simulink model "LQI_example"  (R2023b)
settings: Solver=ode8  StartTime=0.0  StopTime=5  FixedStep=0.04  RelTol=1e-3
values from neighbouring files (symbols this model uses):
  A = [0 1; -2 -3]    [LQI_servo_Example.m]
  B = [0; 1]    [LQI_servo_Example.m]
  K_lqi = lqi( plant, Q, R)    [LQI_servo_Example.m]
settings Model: Creator=afons  LastModifiedBy=afons

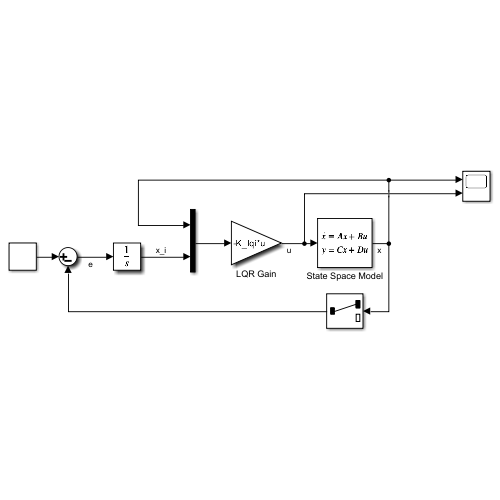
[thumbnail: Simulink's stored preview of the top-level diagram]
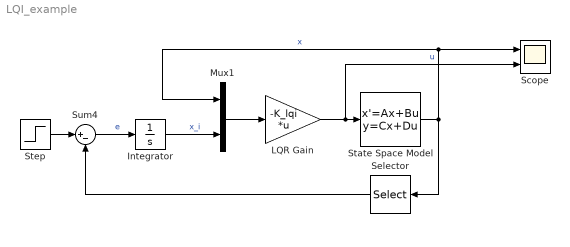
== system LQI_example ==
  Integrator : Integrator
  LQR Gain : Gain  Gain=-K_lqi  Multiplication=Matrix(K*u)  SaturateOnIntegerOverflow=on  OutDataTypeStr=Inherit: Same as input  ParamDataTypeStr=Inherit: Same as input
  Mux1 : Mux  Inputs=2
  Scope : Scope  NumInputPorts=2
  Selector : Selector  InputPortWidth=2  IndexOptions=Index vector (dialog)  Indices=1  OutputSizes=1
  State Space Model : StateSpace  A=A  B=B  C=eye(2)  D=zeros(2,1)  InitialCondition=0
  Step : Step  Time=0  SampleTime=0
  Sum4 : Sum  Inputs=|+-  InputSameDT=on  SaturateOnIntegerOverflow=on  OutDataTypeStr=Inherit: Same as first input
  wires:
  Mux1/1 -> LQR Gain/1
  Integrator/1 -> Mux1/2  "x_i"
  Step/1 -> Sum4/1
  LQR Gain/1 -> Scope/2, State Space Model/1  "u"
  State Space Model/1 -> Selector/1, Mux1/1, Scope/1  "x"
  Sum4/1 -> Integrator/1  "e"
  Selector/1 -> Sum4/2
